simulink model "P4_model"  (R2024b)
settings: Solver=FixedStepAuto  StartTime=0.0  StopTime=240  FixedStep=0.01  RelTol=1e-3
values from neighbouring files (symbols this model uses):
  rps2rpm = 60/(2*pi())    [P4init.m]
  Wp = [transpose(x), transpose(y)]    [GenTrack.m]
undefined symbols (not defined in the file or in its folder): batData, carData, motorData
libraries: slpidlib x2
settings Model: Creator=anshu16  LastModifiedBy=landr
settings SolverCC: AlgebraicLoopSolver=TrustRegion
settings DataIOCC: ReturnWorkspaceOutputs=off
settings OptimizationCC: ReuseModelBlockBuffer=off
settings DebuggingCC: UnconnectedInputMsg=warning  UnconnectedOutputMsg=warning  UnconnectedLineMsg=warning
settings ModelReferenceCC: EnableRefExpFcnMdlSchedulingChecks=on
settings SFSimCC: CustomCodeUndefinedFunction=UseInterfaceOnly
settings RTWCC: GPUComputeCapability=3.5

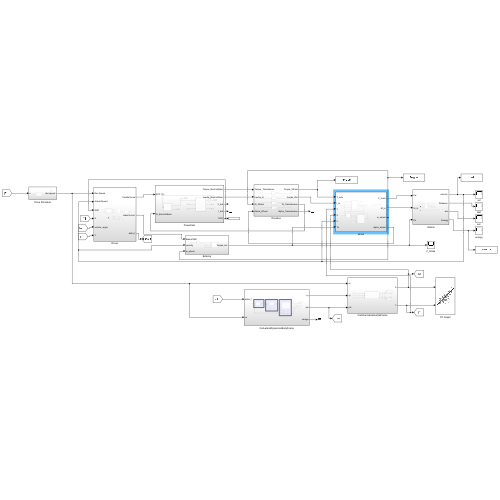
[thumbnail: Simulink's stored preview of the top-level diagram]
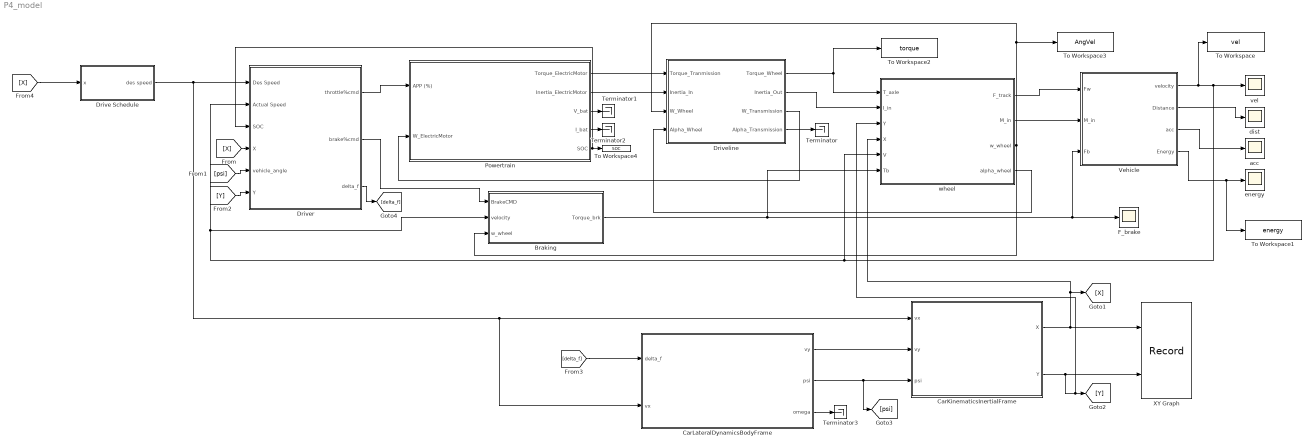
== system P4_model ==
  Braking : Subsystem
  CarKinematicsInertialFrame : Subsystem
  CarLateralDynamicsBodyFrame : Subsystem
  Drive Schedule : Subsystem
  Driveline : Subsystem
  "Driver " : Subsystem
  F_brake : Scope
  Powertrain : Subsystem
  Terminator{,1..3} (4 alike) : Terminator
  To Workspace : ToWorkspace  VariableName=vel  SaveFormat=Timeseries  SampleTime=-1
  To Workspace1 : ToWorkspace  VariableName=energy  SaveFormat=Timeseries  SampleTime=-1
  To Workspace2 : ToWorkspace  VariableName=torque  SaveFormat=Timeseries  SampleTime=-1
  To Workspace3 : ToWorkspace  VariableName=AngVel  SaveFormat=Timeseries  SampleTime=-1
  To Workspace4 : ToWorkspace  VariableName=SOC  SaveFormat=Timeseries  SampleTime=-1
  Vehicle : Subsystem
  XY Graph : Record  FileSettingsInternal="{\"entries\":[{\"content\":{\"excelSettings\":{\"content\":{},\"type\":\"Streamout.ExcelSettings\"}},\"type\":\"Streamout.FileSettingStorage\",\"uuid\":\"\"}],\"packageUris\":[\"http:\\/\\/schema.mathworks.com\\/mf0\\/streamout_blocks\\/R2020a\"],\"version\":\"1.0\"}"  Layout=[1 1]  SignalsInternal="{\"entries\":[{\"content\":{\"signals\":[{\"content\":{\"blockPath\":[],\"dimensions\":[1],\"domain\":\"\",\"lineColor\":\"#a2142f\",\"plots\":[ 1 ],\"port\":1,\"sid\":[\"\"],\"signalID\":1,\"signalName\":\"CarKinematicsInertialFrame:1\"},\"type\":\"RecordBlkView.Signal\",\"uuid\":\"\"},{\"content\":{\"blockPath\":[],\"dimensions\":[1],\"domain\":\"\",\"lineColor\":\"#139fff\",\"plots\":[ 1 ],\"port\":2,\"sid\":[\"\"],\"signalID\":2,\"signalName\":\"CarKinematicsInertialFrame:2\"},\"type\":\"RecordBlkView.Signal\",\"uuid\":\"\"}]},\"type\":\"RecordBlkView.InputSignals\",\"uuid\":\"\"}],\"packageUris\":[\"http:\\/\\/schema.mathworks.com\\/mf0\\/streamout_blocks\\/R2020a\"],\"version\":\"1.0\"}"  VisualizationBindings="{\"xyplotplugin\":{\"info\":[{\"series\":[{\"bindingParametersList\":[{\"parameter\":\"X-Axis\",\"signalID\":1,\"signalName\":\"CarKinematicsInertialFrame:1\"},{\"parameter\":\"Y-Axis\",\"signalID\":2,\"signalName\":\"CarKinematicsInertialFrame:2\"}],\"seriesID\":0}],\"subplotID\":1}]}}"  CompatibilityTag=XY  st=-1
  acc : Scope
  dist : Scope
  energy : Scope
  vel : Scope
  "wheel " : Subsystem
  wires:
  "Driver "/2("brake%cmd ") -> Braking/1("BrakeCMD ")
  Braking/1("Torque_brk ") -> "wheel "/6(Tb), Vehicle/3("Fb "), F_brake/1
  Vehicle/3(acc) -> acc/1
  "wheel "/2(M_in) -> Vehicle/2("M_in ")
  "wheel "/1(F_track) -> Vehicle/1("Fw ")
  Vehicle/2("Distance ") -> dist/1
  Vehicle/1("velocity ") -> To Workspace/1, vel/1, "Driver "/2(Actual Speed), Braking/2("velocity "), "wheel "/5(V)
  "wheel "/4(alpha_wheel) -> Driveline/4(Alpha_Wheel)
  "wheel "/3(w_wheel) -> Driveline/3(W_Wheel), To Workspace3/1, Braking/3(w_wheel)
  Vehicle/4(Energy) -> To Workspace1/1, energy/1
  "Driver "/1(throttle%cmd) -> Powertrain/1(APP (%))
  Powertrain/3(V_bat) -> Terminator1/1
  Powertrain/4(I_bat) -> Terminator2/1
  Powertrain/1(Torque_ElectricMotor) -> Driveline/1(Torque_Tranmission)
  Powertrain/2(Inertia_ElectricMotor) -> Driveline/2(Inertia_In)
  Driveline/3(W_Transmission) -> Powertrain/2(W_ElectricMotor)
  Driveline/4(Alpha_Transmission) -> Terminator/1
  Driveline/2(Inertia_Out) -> "wheel "/2(I_in)
  Driveline/1(Torque_Wheel) -> To Workspace2/1, "wheel "/1(T_axle)
  Powertrain/5(SOC) -> "Driver "/3(SOC), To Workspace4/1
  CarKinematicsInertialFrame/1(X) -> "wheel "/4(X), [X], XY Graph/1
  CarKinematicsInertialFrame/2(Y) -> "wheel "/3(Y), [Y], XY Graph/2
  CarLateralDynamicsBodyFrame/1(vy) -> CarKinematicsInertialFrame/2(vy)
  CarLateralDynamicsBodyFrame/2(psi) -> [psi], CarKinematicsInertialFrame/3(psi)
  Drive Schedule/1("des speed ") -> CarLateralDynamicsBodyFrame/2(vx), CarKinematicsInertialFrame/1(vx), "Driver "/1("Des Speed ")
  [X] -> "Driver "/4(X)
  [psi] -> "Driver "/5(vehicle_angle)
  [Y] -> "Driver "/6(Y)
  "Driver "/3(delta_f) -> [delta_f]
  [delta_f] -> CarLateralDynamicsBodyFrame/1(delta_f)
  CarLateralDynamicsBodyFrame/3(omega) -> Terminator3/1
  [X] -> Drive Schedule/1(x)

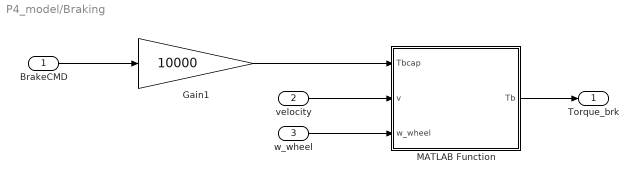
== system P4_model/Braking ==
  "BrakeCMD " : Inport
  "velocity " : Inport  Port=2
  w_wheel : Inport  Port=3
  Gain1 : Gain  Gain=10000
  MATLAB Function : MATLAB Function  TreatAsAtomicUnit=on
  "Torque_brk " : Outport  VectorParamsAs1DForOutWhenUnconnected=off
  wires:
  "BrakeCMD "/1 -> Gain1/1
  Gain1/1 -> MATLAB Function/1(Tbcap)
  MATLAB Function/1(Tb) -> "Torque_brk "/1
  "velocity "/1 -> MATLAB Function/2(v)
  w_wheel/1 -> MATLAB Function/3(w_wheel)

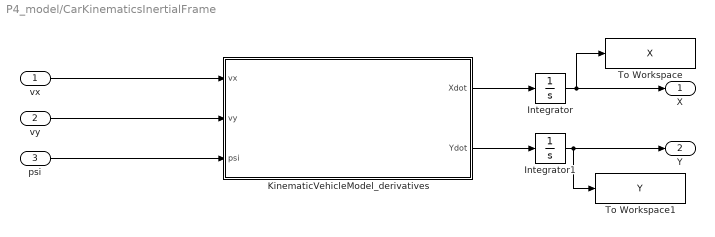
== system P4_model/CarKinematicsInertialFrame ==
  vx : Inport
  vy : Inport  Port=2
  psi : Inport  Port=3
  Integrator : Integrator  InitialCondition=carData.init.X0
  Integrator1 : Integrator  InitialCondition=carData.init.Y0
  KinematicVehicleModel_derivatives : MATLAB Function  TreatAsAtomicUnit=on  mask{obj=carData}
      mask prompts: obj "obj structure"
  To Workspace : ToWorkspace  VariableName=X  SaveFormat=Timeseries  SampleTime=-1
  To Workspace1 : ToWorkspace  VariableName=Y  SaveFormat=Timeseries  SampleTime=-1
  X : Outport
  Y : Outport  Port=2
  wires:
  KinematicVehicleModel_derivatives/1(Xdot) -> Integrator/1
  KinematicVehicleModel_derivatives/2(Ydot) -> Integrator1/1
  Integrator/1 -> To Workspace/1, X/1
  Integrator1/1 -> To Workspace1/1, Y/1
  vx/1 -> KinematicVehicleModel_derivatives/1(vx)
  vy/1 -> KinematicVehicleModel_derivatives/2(vy)
  psi/1 -> KinematicVehicleModel_derivatives/3(psi)

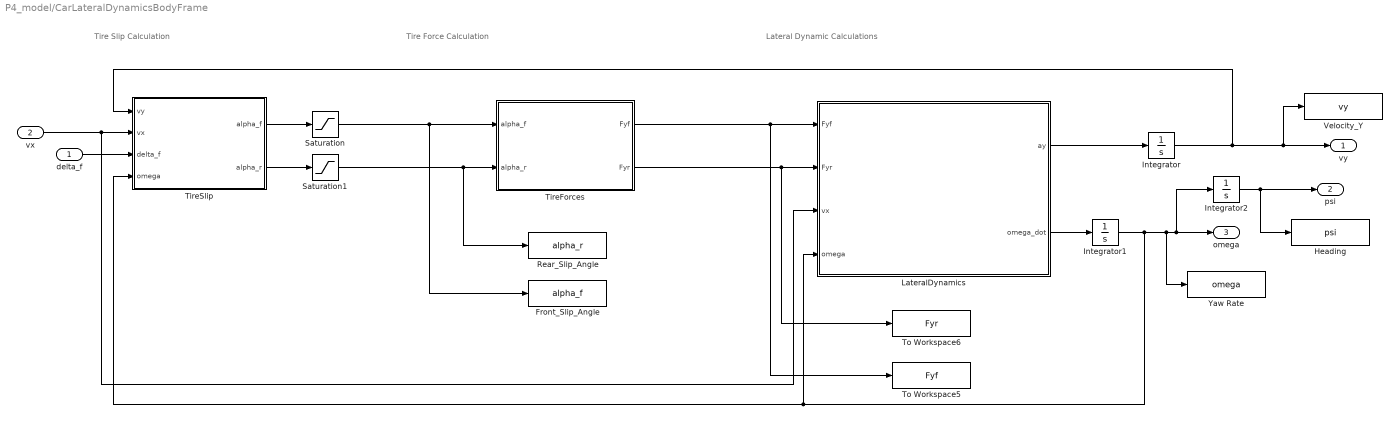
== system P4_model/CarLateralDynamicsBodyFrame ==
  note: Tire Slip Calculation
  note: Tire Force Calculation
  note: Lateral Dynamic Calculations
  delta_f : Inport
  vx : Inport  Port=2
  Front_Slip_Angle : ToWorkspace  VariableName=alpha_f  SaveFormat=Timeseries  SampleTime=-1
  Heading : ToWorkspace  VariableName=psi  SaveFormat=Timeseries  SampleTime=-1
  Integrator : Integrator  InitialCondition=carData.init.vy0
  Integrator1 : Integrator  InitialCondition=carData.init.omega0
  Integrator2 : Integrator  InitialCondition=carData.init.psi0
  LateralDynamics : MATLAB Function  TreatAsAtomicUnit=on  mask{obj=carData}
      mask prompts: obj "obj structure"
  Rear_Slip_Angle : ToWorkspace  VariableName=alpha_r  SaveFormat=Timeseries  SampleTime=-1
  Saturation : Saturate  UpperLimit=carData.maxAlpha  LowerLimit=-carData.maxAlpha
  Saturation1 : Saturate  UpperLimit=carData.maxAlpha  LowerLimit=-carData.maxAlpha
  TireForces : MATLAB Function  TreatAsAtomicUnit=on  mask{obj=carData}
      mask prompts: obj "obj structure"
  TireSlip : MATLAB Function  TreatAsAtomicUnit=on  mask{obj=carData}
      mask prompts: obj "obj structure"
  To Workspace5 : ToWorkspace  VariableName=Fyf  SaveFormat=Timeseries  SampleTime=-1
  To Workspace6 : ToWorkspace  VariableName=Fyr  SaveFormat=Timeseries  SampleTime=-1
  Velocity_Y : ToWorkspace  VariableName=vy  SaveFormat=Timeseries  SampleTime=-1
  Yaw Rate : ToWorkspace  VariableName=omega  SaveFormat=Timeseries  SampleTime=-1
  vy : Outport
  psi : Outport  Port=2
  omega : Outport  Port=3
  wires:
  LateralDynamics/1(ay) -> Integrator/1
  Integrator/1 -> vy/1, Velocity_Y/1, TireSlip/1(vy)
  LateralDynamics/2(omega_dot) -> Integrator1/1
  Integrator1/1 -> Integrator2/1, omega/1, Yaw Rate/1, LateralDynamics/4(omega), TireSlip/4(omega)
  TireSlip/1(alpha_f) -> Saturation/1
  TireSlip/2(alpha_r) -> Saturation1/1
  TireForces/1(Fyf) -> LateralDynamics/1(Fyf), To Workspace5/1
  TireForces/2(Fyr) -> LateralDynamics/2(Fyr), To Workspace6/1
  Saturation/1 -> TireForces/1(alpha_f), Front_Slip_Angle/1
  Saturation1/1 -> TireForces/2(alpha_r), Rear_Slip_Angle/1
  vx/1 -> TireSlip/2(vx), LateralDynamics/3(vx)
  delta_f/1 -> TireSlip/3(delta_f)
  Integrator2/1 -> Heading/1, psi/1

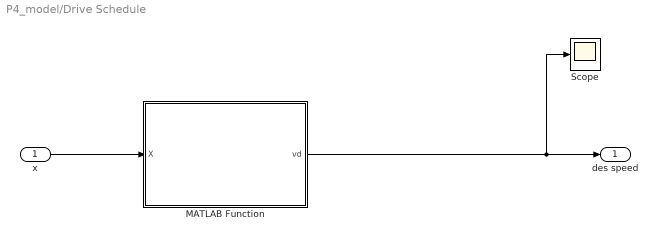
== system P4_model/Drive Schedule ==
  x : Inport
  MATLAB Function : MATLAB Function  TreatAsAtomicUnit=on
  Scope : Scope
  "des speed " : Outport  VectorParamsAs1DForOutWhenUnconnected=off
  wires:
  x/1 -> MATLAB Function/1(X)
  MATLAB Function/1(vd) -> "des speed "/1, Scope/1

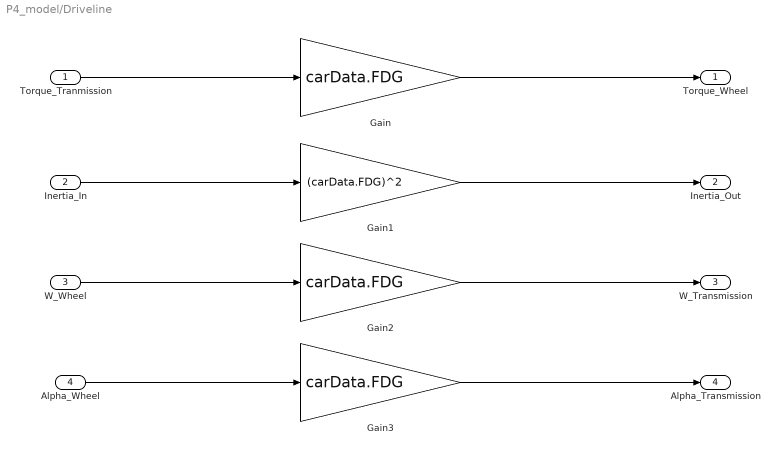
== system P4_model/Driveline ==
  Torque_Tranmission : Inport
  Inertia_In : Inport  Port=2
  W_Wheel : Inport  Port=3
  Alpha_Wheel : Inport  Port=4
  Gain : Gain  Gain=carData.FDG
  Gain1 : Gain  Gain=(carData.FDG)^2
  Gain2 : Gain  Gain=carData.FDG
  Gain3 : Gain  Gain=carData.FDG
  Torque_Wheel : Outport
  Inertia_Out : Outport  Port=2
  W_Transmission : Outport  Port=3
  Alpha_Transmission : Outport  Port=4
  wires:
  Torque_Tranmission/1 -> Gain/1
  Inertia_In/1 -> Gain1/1
  W_Wheel/1 -> Gain2/1
  Alpha_Wheel/1 -> Gain3/1
  Gain/1 -> Torque_Wheel/1
  Gain1/1 -> Inertia_Out/1
  Gain2/1 -> W_Transmission/1
  Gain3/1 -> Alpha_Transmission/1

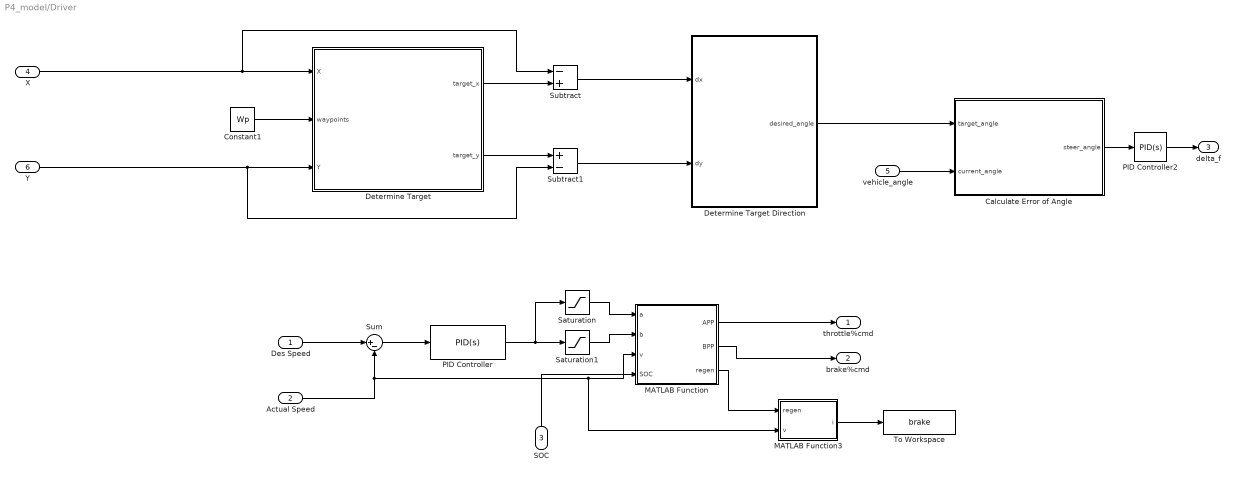
== system P4_model/Driver  ==
  "Des Speed " : Inport
  Actual Speed : Inport  Port=2
  SOC : Inport  Port=3
  X : Inport  Port=4
  vehicle_angle : Inport  Port=5
  Y : Inport  Port=6
  Calculate Error of Angle : MATLAB Function  TreatAsAtomicUnit=on
  Constant1 : Constant  Value=Wp
  Determine Target : MATLAB Function  TreatAsAtomicUnit=on
  Determine Target Direction : MATLAB Function  TreatAsAtomicUnit=on
  MATLAB Function : MATLAB Function  TreatAsAtomicUnit=on
  MATLAB Function3 : MATLAB Function  TreatAsAtomicUnit=on
  PID Controller : slpidlib/PID Controller  Controller=PID  Form=Parallel  TimeDomain=Continuous-time  UseExternalTs=off  SampleTime=-1  IntegratorMethod=Forward Euler  FilterMethod=Forward Euler  ControllerParametersSource=internal  P=0.01  I=0  UseKiTs=off  D=0  UseExternalDerivativeSource=off  N=100  UseFilter=on  TunerSelectOption=Transfer Function Based (PID Tuner App)  InitialConditionSource=internal  InitialConditionForIntegrator=0  InitialConditionForFilter=0  DifferentiatorICPrevScaledInput=0  ExternalReset=none  TrackingMode=off  Kt=1  LimitOutput=on  SatLimitsSource=internal  UpperSaturationLimit=1  LowerSaturationLimit=-1  LinearizeAsGain=off  AntiWindupMode=none  Kb=1  LimitIntegrator=off  UpperIntegratorSaturationLimit=inf  LowerIntegratorSaturationLimit=-inf  POutMin=[]  POutMax=[]  IOutMin=[]  IOutMax=[]  DOutMin=[]  DOutMax=[]  NOutMin=[]  NOutMax=[]  SumOutMin=[]  SumOutMax=[]  SaturationOutMin=[]  SaturationOutMax=[]  PParamMin=[]  PParamMax=[]  IParamMin=[]  IParamMax=[]  DParamMin=[]  DParamMax=[]  NParamMin=[]  NParamMax=[]  KbParamMin=[]  KbParamMax=[]  KtParamMin=[]  KtParamMax=[]  KbOutMin=[]  KbOutMax=[]  KtOutMin=[]  KtOutMax=[]  IntegratorOutMin=[]  IntegratorOutMax=[]  FilterOutMin=[]  FilterOutMax=[]  SumI1OutMin=[]  SumI1OutMax=[]  SumI2OutMin=[]  SumI2OutMax=[]  SumI3OutMin=[]  SumI3OutMax=[]  SumI4OutMin=[]  SumI4OutMax=[]  SumDOutMin=[]  SumDOutMax=[]  DifferentiatorOutMin=[]  DifferentiatorOutMax=[]  FilterDiffOutCoefMin=[]  FilterDiffOutCoefMax=[]  ReciprocalOutMin=[]  ReciprocalOutMax=[]  SumDenOutMin=[]  SumDenOutMax=[]  SumNumOutMin=[]  SumNumOutMax=[]  DivideOutMin=[]  DivideOutMax=[]  UdiffTsProdOutMin=[]  UdiffTsProdOutMax=[]  NTsProdOutMin=[]  NTsProdOutMax=[]  UintegralTsProdOutMin=[]  UintegralTsProdOutMax=[]  UngainTsProdOutMin=[]  UngainTsProdOutMax=[]  ClampingZeroOutDataTypeStr=Inherit: Inherit via back propagation  ClampingZeroOutMin=[]  ClampingZeroOutMax=[]  FilterDenConstantOutDataTypeStr=Inherit: Inherit via back propagation  FilterDenConstantOutMin=[]  FilterDenConstantOutMax=[]  PCopyOutDataTypeStr=Inherit: Inherit via back propagation  PCopyOutMin=[]  PCopyOutMax=[]  NCopyOutDataTypeStr=Inherit: Inherit via back propagation  NCopyOutMin=[]  NCopyOutMax=[]  IntegratorContinuousStateAttributes=''  IntegratorStateMustResolveToSignalObject=off  IntegratorRTWStateStorageClass=Auto  FilterContinuousStateAttributes=''  FilterStateMustResolveToSignalObject=off  FilterRTWStateStorageClass=Auto  ParallelPVariant=InternalParameters  IdealPVariant=Disabled  IVariant=InternalParameters  DVariant=InternalParameters  IntegratorVariant=Continuous  SatVariant=Enabled  AWVariant=Passthrough  PCopyVariant=Disabled  TRVariant=Disabled  FdbkBlocksVariant=Forward  IdealPFdbkVariant=Disabled  SatFdbkVariant=Disabled  DerivativeFilterVariant=ContFilter  NVariant=InternalParameters  NCopyVariant=Disabled  FilterICVariant=InternalICsFilter  IntegratorICVariant=InternalICs  ExternalResetVariant=Disabled  TRSumVariant=Passthrough  SumFdbkVariant=Disabled  SumVariant=Sum_PID  TsampFilterVariant=InternalTs  TsampNgainVariant=Passthrough  TsampIntegralVariant=Disabled_SignalSpec  ExternalSaturationOutDataTypeStr=Inherit: Same as second input  DerivativeSourceVariant=ErrorSignal  PreIntVariant=InternalPreInt
  PID Controller2 : slpidlib/PID Controller  Controller=PID  Form=Parallel  TimeDomain=Continuous-time  UseExternalTs=off  SampleTime=-1  IntegratorMethod=Forward Euler  FilterMethod=Forward Euler  ControllerParametersSource=internal  P=1  I=0.1  UseKiTs=off  D=0  UseExternalDerivativeSource=off  N=100  UseFilter=on  TunerSelectOption=Transfer Function Based (PID Tuner App)  InitialConditionSource=internal  InitialConditionForIntegrator=0  InitialConditionForFilter=0  DifferentiatorICPrevScaledInput=0  ExternalReset=none  TrackingMode=off  Kt=1  LimitOutput=off  SatLimitsSource=internal  UpperSaturationLimit=inf  LowerSaturationLimit=-inf  LinearizeAsGain=on  AntiWindupMode=none  Kb=1  LimitIntegrator=off  UpperIntegratorSaturationLimit=inf  LowerIntegratorSaturationLimit=-inf  POutMin=[]  POutMax=[]  IOutMin=[]  IOutMax=[]  DOutMin=[]  DOutMax=[]  NOutMin=[]  NOutMax=[]  SumOutMin=[]  SumOutMax=[]  SaturationOutMin=[]  SaturationOutMax=[]  PParamMin=[]  PParamMax=[]  IParamMin=[]  IParamMax=[]  DParamMin=[]  DParamMax=[]  NParamMin=[]  NParamMax=[]  KbParamMin=[]  KbParamMax=[]  KtParamMin=[]  KtParamMax=[]  KbOutMin=[]  KbOutMax=[]  KtOutMin=[]  KtOutMax=[]  IntegratorOutMin=[]  IntegratorOutMax=[]  FilterOutMin=[]  FilterOutMax=[]  SumI1OutMin=[]  SumI1OutMax=[]  SumI2OutMin=[]  SumI2OutMax=[]  SumI3OutMin=[]  SumI3OutMax=[]  SumI4OutMin=[]  SumI4OutMax=[]  SumDOutMin=[]  SumDOutMax=[]  DifferentiatorOutMin=[]  DifferentiatorOutMax=[]  FilterDiffOutCoefMin=[]  FilterDiffOutCoefMax=[]  ReciprocalOutMin=[]  ReciprocalOutMax=[]  SumDenOutMin=[]  SumDenOutMax=[]  SumNumOutMin=[]  SumNumOutMax=[]  DivideOutMin=[]  DivideOutMax=[]  UdiffTsProdOutMin=[]  UdiffTsProdOutMax=[]  NTsProdOutMin=[]  NTsProdOutMax=[]  UintegralTsProdOutMin=[]  UintegralTsProdOutMax=[]  UngainTsProdOutMin=[]  UngainTsProdOutMax=[]  ClampingZeroOutDataTypeStr=Inherit: Inherit via back propagation  ClampingZeroOutMin=[]  ClampingZeroOutMax=[]  FilterDenConstantOutDataTypeStr=Inherit: Inherit via back propagation  FilterDenConstantOutMin=[]  FilterDenConstantOutMax=[]  PCopyOutDataTypeStr=Inherit: Inherit via back propagation  PCopyOutMin=[]  PCopyOutMax=[]  NCopyOutDataTypeStr=Inherit: Inherit via back propagation  NCopyOutMin=[]  NCopyOutMax=[]  IntegratorContinuousStateAttributes=''  IntegratorStateMustResolveToSignalObject=off  IntegratorRTWStateStorageClass=Auto  FilterContinuousStateAttributes=''  FilterStateMustResolveToSignalObject=off  FilterRTWStateStorageClass=Auto  ParallelPVariant=InternalParameters  IdealPVariant=Disabled  IVariant=InternalParameters  DVariant=InternalParameters  IntegratorVariant=Continuous  SatVariant=Disabled  AWVariant=Passthrough  PCopyVariant=Disabled  TRVariant=Disabled  FdbkBlocksVariant=Forward  IdealPFdbkVariant=Disabled  SatFdbkVariant=Disabled  DerivativeFilterVariant=ContFilter  NVariant=InternalParameters  NCopyVariant=Disabled  FilterICVariant=InternalICsFilter  IntegratorICVariant=InternalICs  ExternalResetVariant=Disabled  TRSumVariant=Passthrough  SumFdbkVariant=Disabled  SumVariant=Sum_PID  TsampFilterVariant=InternalTs  TsampNgainVariant=Passthrough  TsampIntegralVariant=Disabled_SignalSpec  ExternalSaturationOutDataTypeStr=Inherit: Same as second input  DerivativeSourceVariant=ErrorSignal  PreIntVariant=InternalPreInt
  Saturation : Saturate  UpperLimit=1  LowerLimit=0
  Saturation1 : Saturate  UpperLimit=0  LowerLimit=-1
  Subtract : Sum  Inputs=-+
  Subtract1 : Sum  Inputs=+-
  Sum : Sum  Inputs=|+-
  To Workspace : ToWorkspace  VariableName=brake  SaveFormat=Timeseries  SampleTime=-1
  throttle%cmd : Outport
  "brake%cmd " : Outport  Port=2
  delta_f : Outport  Port=3
  wires:
  "Des Speed "/1 -> Sum/1
  Actual Speed/1 -> MATLAB Function3/2(v), MATLAB Function/3(v), Sum/2
  MATLAB Function/2(BPP) -> "brake%cmd "/1
  MATLAB Function/1(APP) -> throttle%cmd/1
  Sum/1 -> PID Controller/1
  PID Controller/1 -> Saturation/1, Saturation1/1
  Saturation/1 -> MATLAB Function/1(a)
  Saturation1/1 -> MATLAB Function/2(b)
  MATLAB Function/3(regen) -> MATLAB Function3/1(regen)
  SOC/1 -> MATLAB Function/4(SOC)
  Subtract1/1 -> Determine Target Direction/2(dy)
  PID Controller2/1 -> delta_f/1
  Determine Target/2(target_y) -> Subtract1/1
  Constant1/1 -> Determine Target/2(waypoints)
  X/1 -> Subtract/1, Determine Target/1(X)
  Subtract/1 -> Determine Target Direction/1(dx)
  Determine Target Direction/1(desired_angle) -> Calculate Error of Angle/1(target_angle)
  Calculate Error of Angle/1(steer_angle) -> PID Controller2/1
  Determine Target/1(target_x) -> Subtract/2
  Y/1 -> Subtract1/2, Determine Target/3(Y)
  vehicle_angle/1 -> Calculate Error of Angle/2(current_angle)
  MATLAB Function3/1(i) -> To Workspace/1

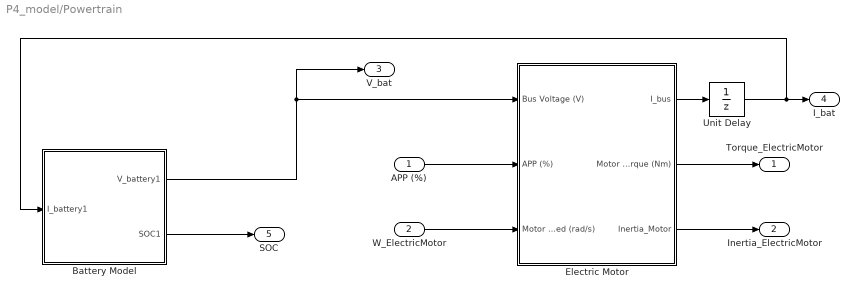
== system P4_model/Powertrain ==
  APP (%) : Inport
  W_ElectricMotor : Inport  Port=2
  Battery Model : Subsystem  TreatAsAtomicUnit=on
  Electric Motor : Subsystem  TreatAsAtomicUnit=on
  Unit Delay : UnitDelay  SampleTime=-1  HasFrameUpgradeWarning=on
  Torque_ElectricMotor : Outport
  Inertia_ElectricMotor : Outport  Port=2
  V_bat : Outport  Port=3
  I_bat : Outport  Port=4
  SOC : Outport  Port=5
  wires:
  Unit Delay/1 -> Battery Model/1(I_battery1), I_bat/1
  Battery Model/2(SOC1) -> SOC/1
  Battery Model/1(V_battery1) -> Electric Motor/1(Bus Voltage (V)), V_bat/1
  Electric Motor/1(I_bus) -> Unit Delay/1
  Electric Motor/2(Motor Torque (Nm)) -> Torque_ElectricMotor/1
  Electric Motor/3(Inertia_Motor) -> Inertia_ElectricMotor/1
  W_ElectricMotor/1 -> Electric Motor/3(Motor Speed (rad/s))
  APP (%)/1 -> Electric Motor/2(APP (%))

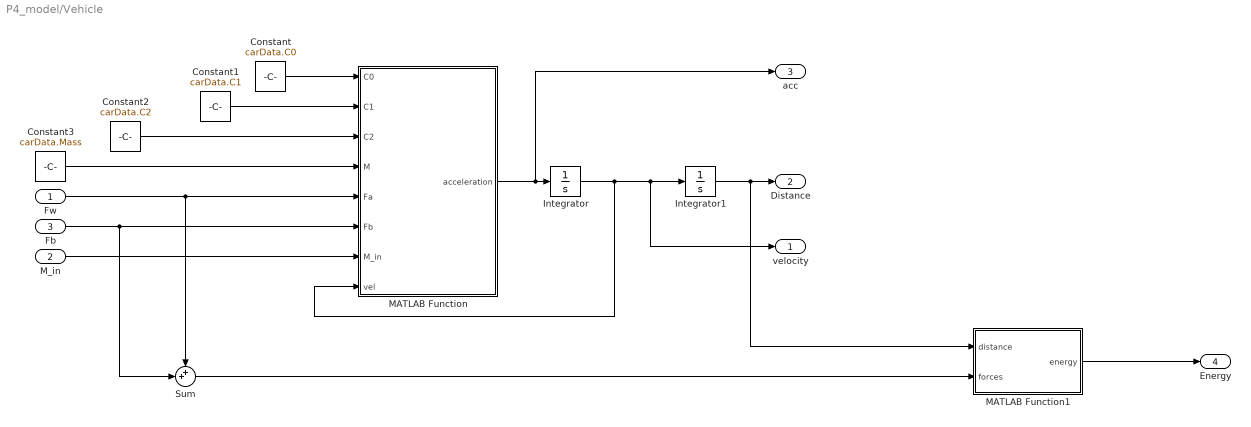
== system P4_model/Vehicle ==
  "Fw " : Inport
  "M_in " : Inport  Port=2
  "Fb " : Inport  Port=3
  Constant : Constant  Value=carData.C0
  Constant1 : Constant  Value=carData.C1
  Constant2 : Constant  Value=carData.C2
  Constant3 : Constant  Value=carData.Mass
  Integrator : Integrator  LimitOutput=on  LowerSaturationLimit=0
  Integrator1 : Integrator
  MATLAB Function : MATLAB Function  TreatAsAtomicUnit=on
  MATLAB Function1 : MATLAB Function  TreatAsAtomicUnit=on
  Sum : Sum  Inputs=++|
  "velocity " : Outport  VectorParamsAs1DForOutWhenUnconnected=off
  "Distance " : Outport  Port=2  VectorParamsAs1DForOutWhenUnconnected=off
  acc : Outport  Port=3
  Energy : Outport  Port=4  VectorParamsAs1DForOutWhenUnconnected=off
  wires:
  Constant1/1 -> MATLAB Function/2(C1)
  Constant/1 -> MATLAB Function/1(C0)
  MATLAB Function/1(acceleration) -> acc/1, Integrator/1
  Constant2/1 -> MATLAB Function/3(C2)
  Constant3/1 -> MATLAB Function/4(M)
  "Fw "/1 -> Sum/1, MATLAB Function/5(Fa)
  "Fb "/1 -> Sum/2, MATLAB Function/6(Fb)
  Integrator/1 -> MATLAB Function/8(vel), "velocity "/1, Integrator1/1
  Integrator1/1 -> MATLAB Function1/1(distance), "Distance "/1
  "M_in "/1 -> MATLAB Function/7(M_in)
  Sum/1 -> MATLAB Function1/2(forces)
  MATLAB Function1/1(energy) -> Energy/1

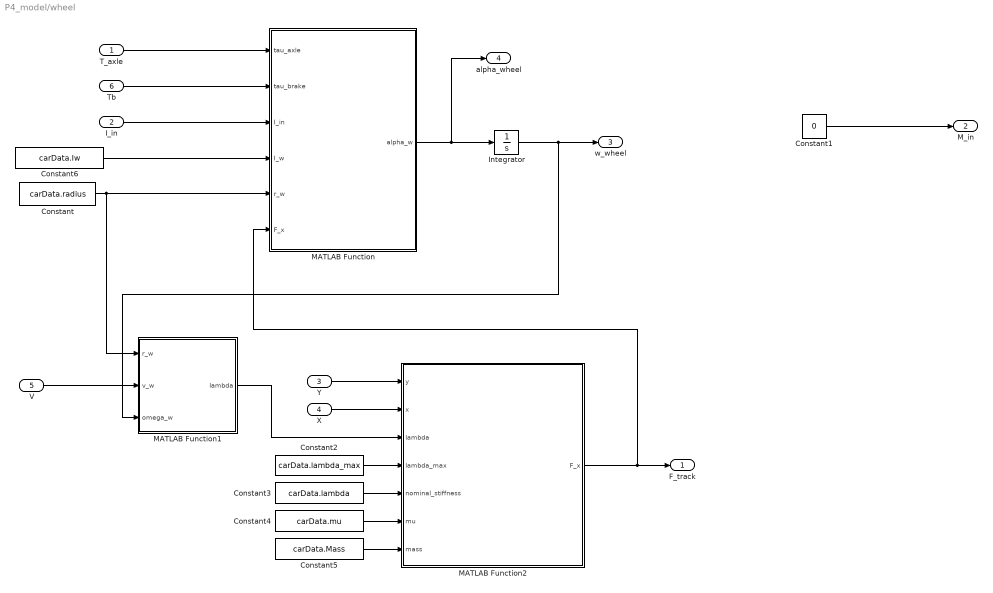
== system P4_model/wheel  ==
  T_axle : Inport
  I_in : Inport  Port=2
  Y : Inport  Port=3
  X : Inport  Port=4
  V : Inport  Port=5
  Tb : Inport  Port=6
  Constant : Constant  Value=carData.radius
  Constant1 : Constant  Value=0
  Constant2 : Constant  Value=carData.lambda_max
  Constant3 : Constant  Value=carData.lambda
  Constant4 : Constant  Value=carData.mu
  Constant5 : Constant  Value=carData.Mass
  Constant6 : Constant  Value=carData.Iw
  Integrator : Integrator
  MATLAB Function : MATLAB Function  TreatAsAtomicUnit=on
  MATLAB Function1 : MATLAB Function  TreatAsAtomicUnit=on
  MATLAB Function2 : MATLAB Function  TreatAsAtomicUnit=on
  F_track : Outport
  M_in : Outport  Port=2
  w_wheel : Outport  Port=3
  alpha_wheel : Outport  Port=4
  wires:
  Constant/1 -> MATLAB Function1/1(r_w), MATLAB Function/5(r_w)
  Tb/1 -> MATLAB Function/2(tau_brake)
  I_in/1 -> MATLAB Function/3(I_in)
  T_axle/1 -> MATLAB Function/1(tau_axle)
  Constant6/1 -> MATLAB Function/4(I_w)
  MATLAB Function/1(alpha_w) -> alpha_wheel/1, Integrator/1
  Integrator/1 -> MATLAB Function1/3(omega_w), w_wheel/1
  Constant1/1 -> M_in/1
  V/1 -> MATLAB Function1/2(v_w)
  MATLAB Function1/1(lambda) -> MATLAB Function2/3(lambda)
  MATLAB Function2/1(F_x) -> MATLAB Function/6(F_x), F_track/1
  Constant2/1 -> MATLAB Function2/4(lambda_max)
  Constant3/1 -> MATLAB Function2/5(nominal_stiffness)
  Constant4/1 -> MATLAB Function2/6(mu)
  Constant5/1 -> MATLAB Function2/7(mass)
  X/1 -> MATLAB Function2/2(x)
  Y/1 -> MATLAB Function2/1(y)

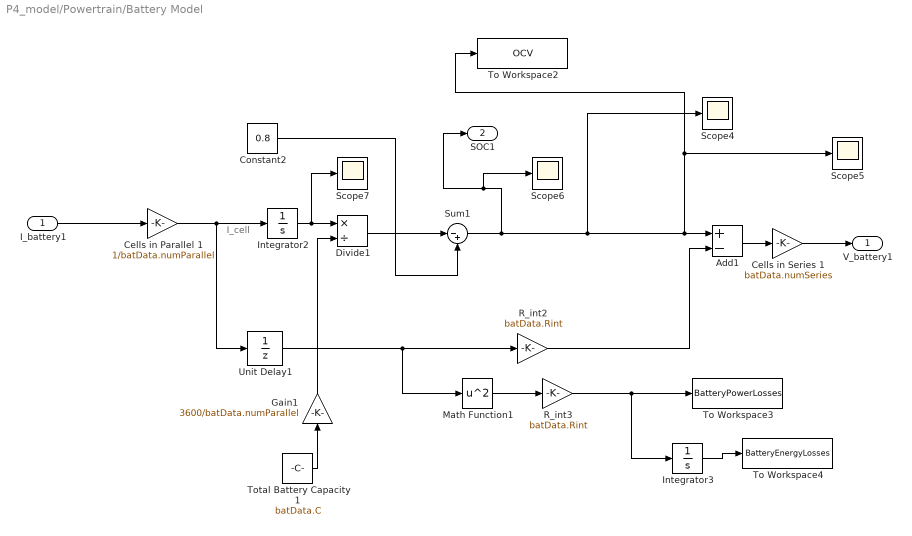
== system P4_model/Powertrain/Battery Model ==
  note: I_cell
  I_battery1 : Inport
  Add1 : Sum  Inputs=+-
  Cells in Parallel 1 : Gain  Gain=1/batData.numParallel
  Cells in Series 1 : Gain  Gain=batData.numSeries
  Constant2 : Constant  Value=0.8
  Divide1 : Product  Inputs=*/
  Gain1 : Gain  Gain=3600/batData.numParallel
  Integrator2 : Integrator
  Integrator3 : Integrator
  Math Function1 : Math  Operator=square
  R_int2 : Gain  Gain=batData.Rint
  R_int3 : Gain  Gain=batData.Rint
  Scope{4..7} (4 alike) : Scope
  Sum1 : Sum  Inputs=|-+
  To Workspace2 : ToWorkspace  VariableName=OCV  SaveFormat=Timeseries  SampleTime=-1
  To Workspace3 : ToWorkspace  VariableName=BatteryPowerLosses  SaveFormat=Timeseries  SampleTime=-1
  To Workspace4 : ToWorkspace  VariableName=BatteryEnergyLosses  SaveFormat=Timeseries  SampleTime=-1
  Total Battery Capacity 1 : Constant  Value=batData.C
  Unit Delay1 : UnitDelay  SampleTime=-1  HasFrameUpgradeWarning=on
  V_battery1 : Outport
  SOC1 : Outport  Port=2
  wires:
  Constant2/1 -> Sum1/2
  I_battery1/1 -> Cells in Parallel 1/1
  Add1/1 -> Cells in Series 1/1
  Math Function1/1 -> R_int3/1
  R_int3/1 -> Integrator3/1, To Workspace3/1
  Cells in Parallel 1/1 -> Unit Delay1/1, Integrator2/1
  Gain1/1 -> Divide1/2
  Divide1/1 -> Sum1/1
  Cells in Series 1/1 -> V_battery1/1
  Sum1/1 -> To Workspace2/1, Scope5/1, Add1/1, Scope4/1, Scope6/1, SOC1/1
  Integrator3/1 -> To Workspace4/1
  Integrator2/1 -> Scope7/1, Divide1/1
  R_int2/1 -> Add1/2
  Unit Delay1/1 -> Math Function1/1, R_int2/1
  Total Battery Capacity 1/1 -> Gain1/1

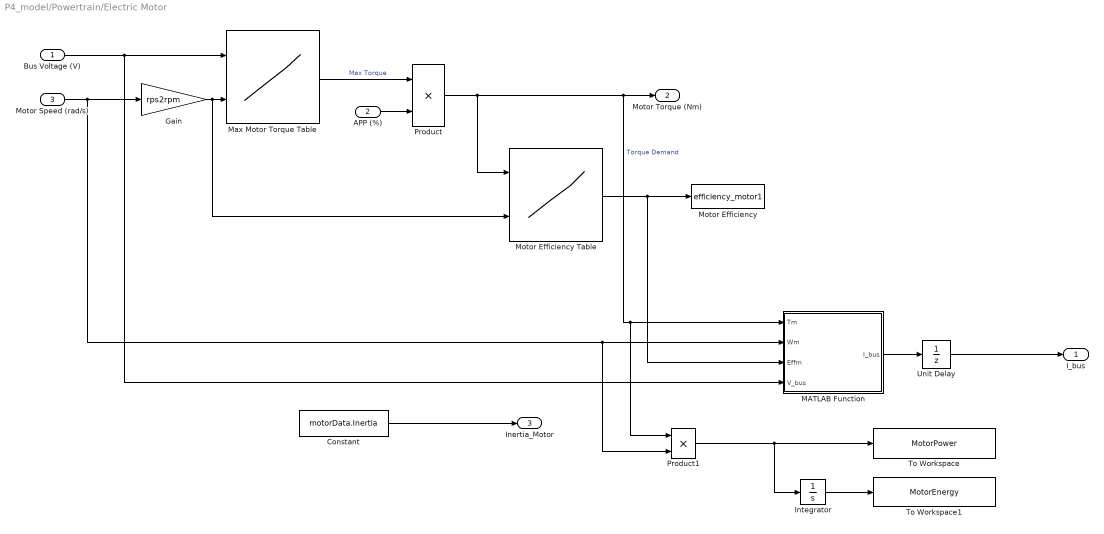
== system P4_model/Powertrain/Electric Motor ==
  Bus Voltage (V) : Inport
  APP (%) : Inport  Port=2
  Motor Speed (rad/s) : Inport  Port=3
  Constant : Constant  Value=motorData.Inertia
  Gain : Gain  Gain=rps2rpm
  Integrator : Integrator
  MATLAB Function : MATLAB Function  TreatAsAtomicUnit=on
  Max Motor Torque Table : Lookup_n-D  BreakpointsForDimension1=motorData.vbus  BreakpointsForDimension2=motorData.rpm  BreakpointsForDimension3=[5, 7]  Table=motorData.maxtorque  InternalRulePriority=Speed  RndMeth=Simplest
      settings: InputPortMap=u0,u1
  Motor Efficiency : ToWorkspace  VariableName=efficiency_motor1  SaveFormat=Timeseries  SampleTime=-1
  Motor Efficiency Table : Lookup_n-D  BreakpointsForDimension1=motorData.eta_torque  BreakpointsForDimension2=motorData.eta_speed  BreakpointsForDimension3=[5, 7]  Table=motorData.eta_val  InternalRulePriority=Speed  RndMeth=Simplest
      settings: InputPortMap=u0,u1
  Product : Product
  Product1 : Product
  To Workspace : ToWorkspace  VariableName=MotorPower  SaveFormat=Timeseries  SampleTime=-1
  To Workspace1 : ToWorkspace  VariableName=MotorEnergy  SaveFormat=Timeseries  SampleTime=-1
  Unit Delay : UnitDelay  SampleTime=-1  HasFrameUpgradeWarning=on
  I_bus : Outport
  Motor Torque (Nm) : Outport  Port=2
  Inertia_Motor : Outport  Port=3
  wires:
  Constant/1 -> Inertia_Motor/1
  APP (%)/1 -> Product/2
  Max Motor Torque Table/1 -> Product/1  "Max Torque"
  Product/1 -> Motor Efficiency Table/1, Product1/1, MATLAB Function/1(Tm), Motor Torque (Nm)/1  "Torque Demand"
  Gain/1 -> Motor Efficiency Table/2, Max Motor Torque Table/2
  Motor Speed (rad/s)/1 -> Gain/1, Product1/2, MATLAB Function/2(Wm)
  Motor Efficiency Table/1 -> MATLAB Function/3(Effm), Motor Efficiency/1
  Integrator/1 -> To Workspace1/1
  Product1/1 -> Integrator/1, To Workspace/1
  MATLAB Function/1(I_bus) -> Unit Delay/1
  Unit Delay/1 -> I_bus/1
  Bus Voltage (V)/1 -> MATLAB Function/4(V_bus), Max Motor Torque Table/1

== matlab function P4_model/CarLateralDynamicsBodyFrame/LateralDynamics ==
  data: Fyf input; Fyr input size=1; vx input; omega input; ay output; obj parameter; omega_dot output
function [ay, omega_dot] = fcn(Fyf, Fyr, vx, omega, obj)

Fy = Fyf + Fyr;
ay = Fy / obj.Mass - omega * vx;
        
M  = Fyf * obj.lf - Fyr * obj.lr;        
omega_dot = M / obj.Inertia;        

end

== matlab function P4_model/CarLateralDynamicsBodyFrame/TireForces ==
  data: alpha_f input; alpha_r input; Fyf output; obj parameter; Fyr output
function [Fyf, Fyr] = fcn(alpha_f, alpha_r, obj)

Fyf = min(obj.Fyfmax,obj.Calpha_f * alpha_f);
Fyr = min(obj.Fyrmax, obj.Calpha_r * alpha_r);
end

== matlab function P4_model/CarLateralDynamicsBodyFrame/TireSlip ==
  data: vy input size=1; vx input; delta_f input size=1; omega input; alpha_f output; obj parameter; alpha_r output
function [alpha_f, alpha_r] = fcn(vy,  vx, delta_f, omega, obj)


if abs(vx)> obj.vx_threshold1
      alpha_f = delta_f - (vy + omega * obj.lf) / vx;
      alpha_r = - (vy - omega * obj.lr) / vx;
else
      alpha_f = 0;
      alpha_r = 0;
end



end

== matlab function P4_model/CarKinematicsInertialFrame/KinematicVehicleModel_derivatives ==
  data: vx input; vy input; psi input size=1; Xdot output; Ydot output
    function [Xdot, Ydot] = fcn(vx, vy, psi)
    temp = TF(psi) * [vx;vy]; 
    Xdot = temp(1);
    Ydot = temp(2);
  
end

function y = TF(psi)
    y = [cos(psi), -sin(psi); sin(psi), cos(psi)];
end

== matlab function P4_model/Driver /Calculate Error of Angle ==
  data: target_angle input; steer_angle output; current_angle input
function steer_angle = diff(target_angle, current_angle)

%steer_angle = angdiff(current_angle, target_angle);
steer_angle = atan2(sin(target_angle - current_angle), cos(target_angle - current_angle));

== matlab function P4_model/Driver /MATLAB Function ==
  data: a input; APP output; BPP output; b input; v input; regen output; SOC input
function [APP,BPP,regen] = fcn(a,b,v, SOC)
if v < (5*(1600/3600))
    regen = 0;
    friction = 1;
    APP = a + b*regen;
    BPP = b*friction;
elseif v == (25*(1600/3600))
    regen = 0.95;
    friction = 0.05;
    APP = a + b*regen;
    BPP = b*friction;
elseif v > (25*(1600/3600))
    regen = 0.95;
    friction = 0.05;
    APP = a + b*regen;
    BPP = b*friction;
else
    regen = (0.95/20)*v*(1600/3600);
    friction = 1 - regen;
    APP = a + b*regen;
    BPP = b*friction;
end

if SOC <= 0.1
    APP = 0;
    BPP = 0;
    regen = 0;
end

== matlab function P4_model/Driver /Determine Target ==
  data: X input; waypoints input; Y input; target_x output; target_y output
function [target_x, target_y] = Driver(X, waypoints, Y)

waypoints = waypoints(1:end-1,:);

% Determine which waypoint is the closest
dist_from_waypoints_sqr = (waypoints(:,1)-X).^2+(waypoints(:,2)-Y).^2;
dist_from_waypoints = sqrt(dist_from_waypoints_sqr);

[~, idx] = min(dist_from_waypoints);

% Look ahead a few waypoints
target_idx = idx + 1;
if target_idx >= height(waypoints)
   target_idx = 1;
end
target_x = waypoints(target_idx,1);
target_y = waypoints(target_idx,2);

== matlab function P4_model/Drive Schedule/MATLAB Function ==
  data: X input; vd output
function vd = fcn(X)

%Vertical Speed
if X > 0 && X < 900
    vd = 67;
%Speed in the Curve
else
    vd = 20;
end

== matlab function P4_model/Driver /MATLAB Function3 ==
  data: regen input; i output; v input
function i = fcn(regen, v)
    speed = v * (3600 / 1600);
    if speed < 5
        regen_i = 0;
        if abs(regen - regen_i) < 1e-6
            i = 0;
        else
            i = 1;
        end

    elseif speed == 25
        regen_i = 0.95;
        if abs(regen - regen_i) < 1e-6
            i = 0;
        else
            i = 1;
        end

    elseif speed > 25
        regen_i = 0.95;
        if abs(regen - regen_i) < 1e-6
            i = 0;
        else
            i = 1;
        end
    else
        regen_i = (0.95/20)*speed - 0.2375;
        if abs(regen - regen_i) < 1e-6
            i = 0;
        else
            i = 1;
        end 
    end

== matlab function P4_model/Driver /Determine Target Direction ==
  data: dx input; desired_angle output; dy input
function desired_angle = fcn(dx,dy)

desired_angle = atan2(dy,dx);

% Make desired_angle a positive value always
if desired_angle < 0
    desired_angle = desired_angle + 2 * pi;
end

== matlab function P4_model/Vehicle/MATLAB Function ==
  data: C0 input; acceleration output; C1 input; C2 input; M input; Fa input; Fb input; M_in input; vel input
function acceleration   = vehicle(C0,C1,C2,M,Fa,Fb,M_in, vel)

acceleration = (((Fa-Fb))-(C0+ C1*vel + C2*(vel)^2))/(M+M_in);

% Fa: Force from wheel
% Fb: Force from brake
% -(C0+ C1*vel + C2*(vel)^2)): Force from drag (opposite direction of motion)

== matlab function P4_model/Vehicle/MATLAB Function1 ==
  data: distance input; forces input; energy output
function energy = fcn(distance,forces)

energy = dot(forces,distance);

== matlab function P4_model/Powertrain/Electric Motor/MATLAB Function ==
  data: Tm input; I_bus output; Wm input; Effm input; V_bus input
function I_bus = fcn(Tm,Wm,Effm,V_bus)
Pm=Tm*Wm;
sgnPm = Pm/(abs(Pm)+0.001);
Pe = Pm/(abs(Effm)^sgnPm);
if V_bus > 1
    I_bus = Pe/V_bus;
else
    I_bus = 0;
end 


%I_bus = ( (Pm) * (Effm)^(sgnPm) ) / V_bus;

== matlab function P4_model/wheel /MATLAB Function ==
  data: tau_axle input; alpha_w output; tau_brake input; I_in input; I_w input; r_w input; F_x input
function alpha_w = wheel_acceleration(tau_axle, tau_brake, I_in, I_w, r_w, F_x)

alpha_w = (tau_axle - tau_brake - F_x * r_w) / (I_in + I_w);

== matlab function P4_model/wheel /MATLAB Function1 ==
  data: r_w input; lambda output; v_w input; omega_w input
function lambda = tire_slip_ratio(r_w, v_w, omega_w)

 % Calculate the effective wheel speed (linear speed equivalent)
    wheel_speed = r_w * omega_w;

    % Use the maximum of the two speeds as the denominator to avoid division by zero
    denom = max(wheel_speed,v_w);

    % If both speeds are zero, define the slip ratio as zero
    if denom == 0
        lambda = 0;
    else
        lambda = (wheel_speed - v_w) / denom;
    end

end

== matlab function P4_model/Braking/MATLAB Function ==
  data: Tbcap input; Tb output; v input; w_wheel input
function Tb = fcn(Tbcap, v, w_wheel)
Tb = Tbcap * v/(abs(v)+0.001);
end

== matlab function P4_model/wheel /MATLAB Function2 ==
  data: y input; x input; lambda input; F_x output; lambda_max input; nominal_stiffness input; mu input; mass input
function F_x = tire_tractive_force(y, x, lambda, lambda_max, nominal_stiffness, mu, mass)
g = 9.81;

if x<0 || x>900 %both curved sections, regular normal force
    N = mass * g/4;

elseif x>=0 && x<=900 && y==0 %bottom straightaway, takes angle into consideration
    N = mass * g*atan(10/900)/4;

elseif x>=0 && x<=900 && y==400 %top straightaway (car is going down, negative slope)
    N = mass * g*-atan(10/900)/4;

else
    N = mass*g/4;
end

C_lambda = nominal_stiffness * mu* N;
if lambda >= 0 
    F_x = C_lambda * min(lambda_max, lambda);
else 
    F_x = C_lambda * max(-lambda_max, lambda);
end
